simulink model "youBot_dynamics_id_alone"  (R2020b)
settings: Solver=VariableStepAuto  StartTime=0.0  StopTime=10.0  RelTol=1e-3
values from neighbouring files (symbols this model uses):
  dth0 = [0; 0; 0]    [dynamic_simulation.m]    (also in init_dynamic_sim.m = dq0)
  dv = 1e-2    (= 0.01)    [Fs_3DOF.m]    (also in init_dynamic_sim.m = 0.001)
  Fc = Fs    [Fs_3DOF.m]    (also in init_dynamic_sim.m)
  Fs = zeros(3,1)    [DynModel_3DOF.m]    (also in Fs_3DOF.m = [0.97571; 0.65131; 0.25819]; InvDynModel_3DOF.m; init_dynamic_sim.m = [0.9, 1.3, 0.5])
  Fv = zeros(3,3)    [DynModel_3DOF.m]    (also in InvDynModel_3DOF.m; init_dynamic_sim.m = diag([0.5,0.37,0.7]))
  nu = nu.*eye(3)    [DynModel_3DOF.m]    (also in InvDynModel_3DOF.m; init_dynamic_sim.m = [0.8554; 0.5780; 0.9997])
  tau_0 = [1.0050; 0.6119; 0.8268]    [init_dynamic_sim.m]
  th0 = 0    [DGM_youBot.m]    (also in DGM_youBot_sym.m; dynamic_simulation.m = q_dh - (q0_kuka - q_rob); init_dynamic_sim.m = theta_DH(2:4) - (q0 - KUKA_offset(2:4)))
  thmax = theta_DH - (qmin - KUKA_offset)    [init_dynamic_sim.m]
  thmin = theta_DH - (qmax - KUKA_offset)    [init_dynamic_sim.m]
libraries: simulink x1
settings Model: Creator=fortineau_vin  LastModifiedBy=fortineau_vin

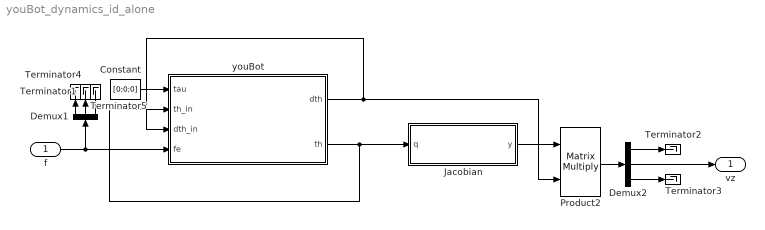
== system youBot_dynamics_id_alone ==
  f : Inport  PortDimensions=3
  Constant : Constant  Value=[0;0;0]
  Demux1 : Demux  Outputs=3
  Demux2 : Demux  Outputs=3
  Jacobian : MATLAB Function  TreatAsAtomicUnit=on
  Product2 : Product  Multiplication=Matrix(*)
  Terminator{1..5} (5 alike) : Terminator
  youBot : Subsystem
  vz : Outport  VectorParamsAs1DForOutWhenUnconnected=off
  wires:
  Demux2/3 -> Terminator3/1
  youBot/1(dth) -> youBot/3(dth_in), Product2/2
  Demux2/2 -> vz/1
  Product2/1 -> Demux2/1
  youBot/2(th) -> youBot/2(th_in), Jacobian/1(q)
  Jacobian/1(y) -> Product2/1
  Demux2/1 -> Terminator2/1
  Constant/1 -> youBot/1(tau)
  Demux1/3 -> Terminator5/1
  Demux1/1 -> Terminator4/1
  Demux1/2 -> Terminator1/1
  f/1 -> Demux1/1, youBot/4(fe)

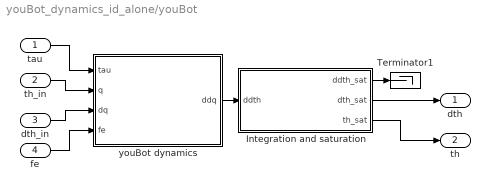
== system youBot_dynamics_id_alone/youBot ==
  tau : Inport
  th_in : Inport  Port=2
  dth_in : Inport  Port=3
  fe : Inport  Port=4
  Integration and saturation : Subsystem
  Terminator1 : Terminator
  youBot dynamics : Subsystem
  dth : Outport  VectorParamsAs1DForOutWhenUnconnected=off
  th : Outport  Port=2  VectorParamsAs1DForOutWhenUnconnected=off
  wires:
  tau/1 -> youBot dynamics/1(tau)
  youBot dynamics/1(ddq) -> Integration and saturation/1(ddth)
  dth_in/1 -> youBot dynamics/3("dq ")
  th_in/1 -> youBot dynamics/2("q ")
  fe/1 -> youBot dynamics/4(fe)
  Integration and saturation/3(th_sat) -> th/1
  Integration and saturation/2(dth_sat) -> dth/1
  Integration and saturation/1(ddth_sat) -> Terminator1/1

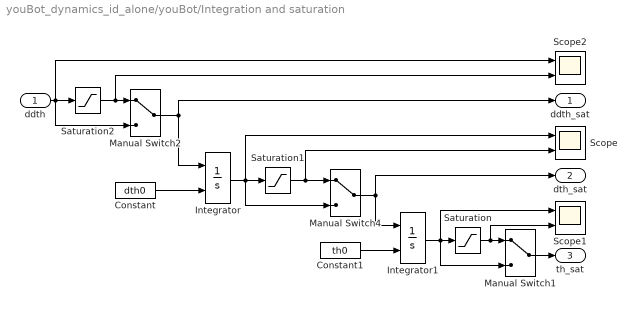
== system youBot_dynamics_id_alone/youBot/Integration and saturation ==
  ddth : Inport
  Constant : Constant  Value=dth0
  Constant1 : Constant  Value=th0
  Integrator : Integrator  InitialConditionSource=external
  Integrator1 : Integrator  InitialConditionSource=external
  Manual Switch1 : ManualSwitch
  Manual Switch2 : ManualSwitch
  Manual Switch4 : ManualSwitch
  Saturation : Saturate  UpperLimit=thmax(2:4)'  LowerLimit=thmin(2:4)'
  Saturation1 : Saturate  UpperLimit=[2.685122; 4.188790; 5.899705]  LowerLimit=[-2.685122; -4.188790; -5.899705]
  Saturation2 : Saturate  UpperLimit=[10;10;10]  LowerLimit=[-10;-10;-10]
  Scope : Scope  NumInputPorts=2
  Scope1 : Scope  NumInputPorts=2
  Scope2 : Scope  NumInputPorts=2
  ddth_sat : Outport  VectorParamsAs1DForOutWhenUnconnected=off
  dth_sat : Outport  Port=2  VectorParamsAs1DForOutWhenUnconnected=off
  th_sat : Outport  Port=3  VectorParamsAs1DForOutWhenUnconnected=off
  wires:
  Manual Switch2/1 -> ddth_sat/1, Integrator/1
  Manual Switch1/1 -> th_sat/1
  Manual Switch4/1 -> Integrator1/1, dth_sat/1
  ddth/1 -> Scope2/1, Manual Switch2/2, Saturation2/1
  Saturation2/1 -> Scope2/2, Manual Switch2/1
  Saturation1/1 -> Scope/2, Manual Switch4/1
  Saturation/1 -> Scope1/2, Manual Switch1/1
  Constant/1 -> Integrator/2
  Integrator/1 -> Scope/1, Manual Switch4/2, Saturation1/1
  Integrator1/1 -> Scope1/1, Manual Switch1/2, Saturation/1
  Constant1/1 -> Integrator1/2

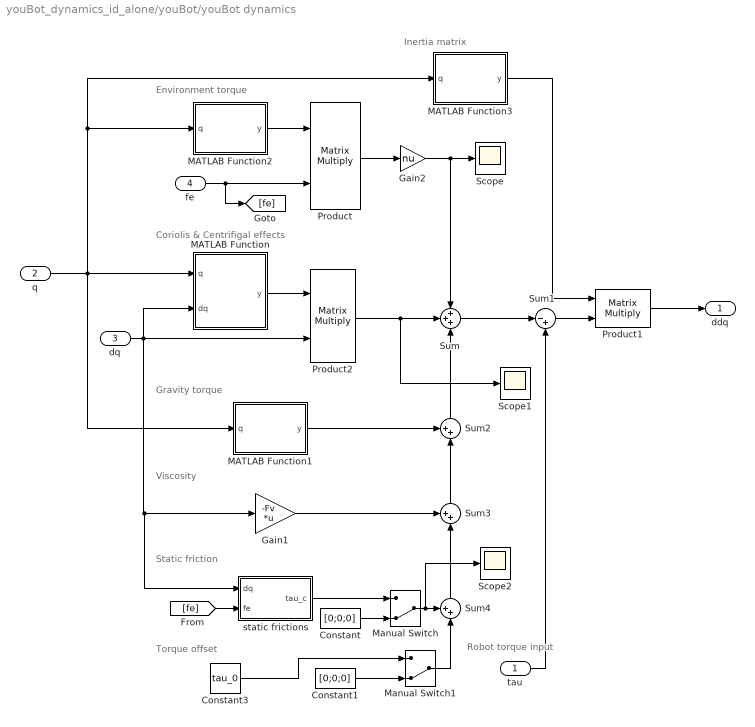
== system youBot_dynamics_id_alone/youBot/youBot dynamics ==
  note: Coriolis & Centrifigal effects
  note: Gravity torque
  note: Environment torque
  note: Robot torque input
  note: Inertia matrix
  note: Viscosity
  note: Static friction
  note: Torque offset
  tau : Inport
  "q " : Inport  Port=2
  "dq " : Inport  Port=3
  fe : Inport  Port=4
  Constant : Constant  Value=[0;0;0]
  Constant1 : Constant  Value=[0;0;0]
  Constant3 : Constant  Value=tau_0
  Gain1 : Gain  Gain=-Fv  Multiplication=Matrix(K*u)
  Gain2 : Gain  Gain=nu
  MATLAB Function : MATLAB Function  TreatAsAtomicUnit=on
  MATLAB Function1 : MATLAB Function  TreatAsAtomicUnit=on
  MATLAB Function2 : MATLAB Function  TreatAsAtomicUnit=on
  MATLAB Function3 : MATLAB Function  TreatAsAtomicUnit=on
  Manual Switch : ManualSwitch  CurrentSetting=0
  Manual Switch1 : ManualSwitch  CurrentSetting=0
  Product : Product  Multiplication=Matrix(*)
  Product1 : Product  Multiplication=Matrix(*)
  Product2 : Product  Multiplication=Matrix(*)
  Scope : Scope
  Scope1 : Scope
  Scope2 : Scope
  Sum : Sum  Inputs=+++
  Sum1 : Sum  Inputs=|-+
  Sum2 : Sum  Inputs=++|
  Sum3 : Sum  Inputs=++|
  Sum4 : Sum  Inputs=++|
  static frictions : Subsystem
  ddq : Outport  VectorParamsAs1DForOutWhenUnconnected=off
  wires:
  "q "/1 -> MATLAB Function3/1(q), MATLAB Function2/1(q), MATLAB Function1/1(q), MATLAB Function/1(q)
  Product/1 -> Gain2/1
  Product1/1 -> ddq/1
  Sum/1 -> Sum1/1
  tau/1 -> Sum1/2
  Product2/1 -> Scope1/1, Sum/2
  MATLAB Function/1(y) -> Product2/1
  MATLAB Function2/1(y) -> Product/1
  MATLAB Function3/1(y) -> Product1/1
  Sum1/1 -> Product1/2
  Gain2/1 -> Sum/1, Scope/1
  MATLAB Function1/1(y) -> Sum2/1
  Sum2/1 -> Sum/3
  [fe] -> static frictions/2(fe)
  "dq "/1 -> static frictions/1(dq), Gain1/1, Product2/2, MATLAB Function/2(dq)
  Sum3/1 -> Sum2/2
  Gain1/1 -> Sum3/1
  static frictions/1(tau_c) -> Manual Switch/1
  Constant/1 -> Manual Switch/2
  fe/1 -> Product/2, [fe]
  Sum4/1 -> Sum3/2
  Manual Switch/1 -> Scope2/1, Sum4/1
  Manual Switch1/1 -> Sum4/2
  Constant3/1 -> Manual Switch1/1
  Constant1/1 -> Manual Switch1/2

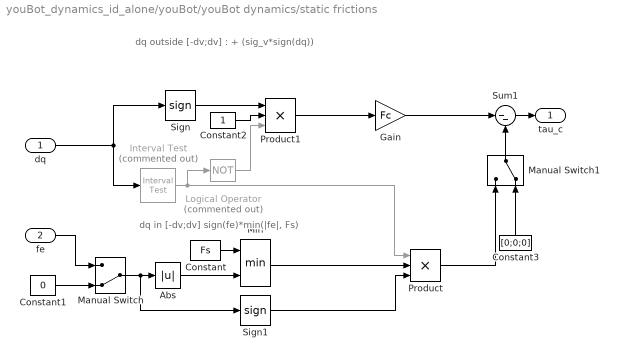
== system youBot_dynamics_id_alone/youBot/youBot dynamics/static frictions ==
  note: dq in [-dv;dv]
      |
      | sign(fe)*min(|fe|, Fs)
  note: dq outside [-dv;dv] : + (sig_v*sign(dq))
  dq : Inport
  fe : Inport  Port=2
  Abs : Abs
  Constant : Constant  Value=Fs
  Constant1 : Constant  Value=0
  Constant2 : Constant
  Constant3 : Constant  Value=[0;0;0]
  Gain : Gain  Gain=Fc
  Interval Test : simulink/Logic and Bit Operations/Interval Test  Commented=on  IntervalClosedRight=on  uplimit=dv  IntervalClosedLeft=on  lowlimit=-dv  OutDataTypeStr=boolean
  Logical Operator : Logic  Commented=on  Operator=NOT  AllPortsSameDT=off  OutDataTypeStr=boolean
  Manual Switch : ManualSwitch  CurrentSetting=0
  Manual Switch1 : ManualSwitch  CurrentSetting=0
  Min : MinMax  Inputs=2
  Product : Product  Inputs=3
  Product1 : Product  Inputs=3
  Sign : Signum
  Sign1 : Signum
  Sum1 : Sum  Inputs=|--
  tau_c : Outport  VectorParamsAs1DForOutWhenUnconnected=off
  wires:
  Sum1/1 -> tau_c/1
  Interval Test/1 -> Logical Operator/1, Product/1
  Abs/1 -> Min/2
  Constant/1 -> Min/1
  Min/1 -> Product/2
  Sign1/1 -> Product/3
  Logical Operator/1 -> Product1/3
  dq/1 -> Sign/1, Interval Test/1
  Product1/1 -> Gain/1
  Gain/1 -> Sum1/1
  Sign/1 -> Product1/1
  Constant1/1 -> Manual Switch/2
  fe/1 -> Manual Switch/1
  Manual Switch/1 -> Sign1/1, Abs/1
  Product/1 -> Manual Switch1/1
  Manual Switch1/1 -> Sum1/2
  Constant3/1 -> Manual Switch1/2
  Constant2/1 -> Product1/2

== matlab function youBot_dynamics_id_alone/youBot/youBot dynamics/MATLAB Function ==
  data: q input; y output; dq input
function y = C_sim(q,dq)
q2 = q(2);
q3 = q(3);
dq1 = dq(1);
dq2 = dq(2);
dq3 = dq(3);
y = C_3DOF(dq1,dq2,dq3,q2,q3);

== matlab function youBot_dynamics_id_alone/youBot/youBot dynamics/MATLAB Function2 ==
  data: q input; y output
function y = tJ_sim(q)
q1 = q(1);
q2 = q(2);
q3 = q(3);
y = J0E_3DOF(q1,q2,q3)';

== matlab function youBot_dynamics_id_alone/youBot/youBot dynamics/MATLAB Function3 ==
  data: q input; y output
function y = iM_sim(q)
q2 = q(2);
q3 = q(3);
y = iM_3DOF(q2,q3);

== matlab function youBot_dynamics_id_alone/Jacobian ==
  data: q input; y output
function y = J(q)
q1 = q(1);
q2 = q(2);
q3 = q(3);
y = J0E_3DOF(q1,q2,q3);

== matlab function youBot_dynamics_id_alone/youBot/youBot dynamics/MATLAB Function1 ==
  data: q input; y output
function y = G_sim(q)
q1 = q(1);
q2 = q(2);
q3 = q(3);
y = G_3DOF(q1,q2,q3);
